simulink model "Model_6DOF_2021a"  (R2021b)
settings: Solver=FixedStepAuto  StartTime=0.0  StopTime=Tfin  FixedStep=0.05  RelTol=1e-3
values from neighbouring files (symbols this model uses):
  adap = 1    [ctrl_mode_param.m]
  Ba_0 = [0 0 0 0 0 0]    [ctrl_mode_param.m]
  Bv_0 = [tgt_speed 0 0 0 0 0]    [ctrl_mode_param.m]
  Bx_0 = [0 0 tgt_depth 0 0 0]    [ctrl_mode_param.m]
  check_angle = 10    [ctrl_mode_param.m]
  Cp = [Cpx' ; Cpy' ; Cpz']    [ctrl_mode_param.m]
  Cp_prime = Cp*Dm    [ctrl_mode_param.m]
  ctrl_mode = 5    [run.m]
  dX_imposed = 10    [ctrl_mode_param.m]
  Seastate = 5    [ctrl_mode_param.m]    (also in run.m = 0)
  tgt_depth = -50    [ctrl_mode_param.m]
  tgt_pitch = 0    [ctrl_mode_param.m]
  tgt_speed = -5    [ctrl_mode_param.m]
  tgt_sway = 0    [ctrl_mode_param.m]
  tgt_yaw = 0    [ctrl_mode_param.m]
undefined symbols (not defined in the file or in its folder): Bb, dA_BP1, dA_BP2, dA_Hull, dA_PH, dA_Sail, dA_SProot, dA_X1a, dA_X1b, dA_X2a, dA_X2b, dA_X3a, dA_X3b, dA_X4a, dA_X4b, Ixx, Ixy, Ixz, Iyy, Iyz, Izz, Mb, n_BP1, n_BP2, n_Hull, n_PH, n_Sail, n_SProot, n_X2a, n_X2b, n_X3a, n_X4a, n_X4b, nt_BP1, nt_BP2, nt_Hull, nt_PH, nt_Sail, nt_SProot, nt_X1a, nt_X1b, nt_X2a, nt_X2b, nt_X3a, nt_X3b, nt_X4a, nt_X4b, vt1_BP1, vt1_BP2, vt1_Hull, vt1_PH, vt1_Sail, vt1_SProot, vt1_X1a, vt1_X1b, vt1_X2a, vt1_X2b, vt1_X3a, vt1_X3b, vt1_X4a ... (+36)
libraries: simulink x19
(part 3 of 6)

== system Model_6DOF_2021a/HDM/HDM B3/M/Mdxi ==
  dX : Inport
  z : Inport  Port=2
  Demux6 : Demux  Outputs=5
  Gain{,1..4} (5 alike) : Gain
  Mux : Mux  Inputs=5
  ZudX1 q+1 : Lookup_n-D  BreakpointsForDimension1=[-30 -20 -10 0 10 20 30]  BreakpointsForDimension2=[-35.0624 -15.3724 -13.8724]  BreakpointsForDimension3=[-5.14444 -3.08666664 -1.54332]  Table=|  InternalRulePriority=Speed  RndMeth=Simplest  InputSameDT=on
      | reshape([0.000594819
      | 0.000394915
      | 0.000195011
      | -4.89222E-06
      | -0.000204796
      | -0.0004047
      | -0.000604603
      | 0.000596203
      | 0.000392018
      | 0.000187833
      | -1.6352E-05
      | -0.000220537
      | -0.000424722
      | -0.000628907
      | 0.000582351
      | 0.000381446
      | 0.000180542
      | -2.03625E-05
      | -0.000221267
      | -0.000422171
      | -0.000623076
      | ],[7,3])
      settings: InputPortMap=u0,u1
  ZudX1 q+2 : Lookup_n-D  BreakpointsForDimension1=[-30 -20 -10 0 10 20 30]  BreakpointsForDimension2=[-35.0624 -15.3724 -13.8724]  BreakpointsForDimension3=[-5.14444 -3.08666664 -1.54332]  Table=|  InternalRulePriority=Speed  RndMeth=Simplest  InputSameDT=on
      | reshape([0.000583784
      | 0.000394316
      | 0.000204847
      | 1.53782E-05
      | -0.000174091
      | -0.000363559
      | -0.000553028
      | 0.00056228
      | 0.000374724
      | 0.000187169
      | -3.86644E-07
      | -0.000187942
      | -0.000375498
      | -0.000563053
      | 0.000546298
      | 0.000362052
      | 0.000177806
      | -6.43933E-06
      | -0.000190685
      | -0.000374931
      | -0.000559176],[7,3])
      settings: InputPortMap=u0,u1
  ZudX1 q+3 : Lookup_n-D  BreakpointsForDimension1=[-30 -20 -10 0 10 20 30]  BreakpointsForDimension2=[-35.0624 -15.3724 -13.8724]  BreakpointsForDimension3=[-5.14444 -3.08666664 -1.54332]  Table=|  InternalRulePriority=Speed  RndMeth=Simplest  InputSameDT=on
      | reshape([-0.000586989
      | -0.000395541
      | -0.000204094
      | -1.26467E-05
      | 0.000178801
      | 0.000370248
      | 0.000561695
      | -0.000568868
      | -0.000379268
      | -0.000189669
      | -6.86388E-08
      | 0.000189531
      | 0.000379131
      | 0.000568731
      | -0.000565299
      | -0.000378949
      | -0.000192598
      | -6.24776E-06
      | 0.000180103
      | 0.000366453
      | 0.000552804],[7,3])
      settings: InputPortMap=u0,u1
  ZudX1 q+4 : Lookup_n-D  BreakpointsForDimension1=[-30 -20 -10 0 10 20 30]  BreakpointsForDimension2=[-35.0624 -15.3724 -13.8724]  BreakpointsForDimension3=[-5.14444 -3.08666664 -1.54332]  Table=|  InternalRulePriority=Speed  RndMeth=Simplest  InputSameDT=on
      | reshape([-0.000638396
      | -0.000426715
      | -0.000215035
      | -3.35454E-06
      | 0.000208326
      | 0.000420006
      | 0.000631687
      | -0.000598951
      | -0.000393944
      | -0.000188937
      | 1.60698E-05
      | 0.000221077
      | 0.000426084
      | 0.000631091
      | -0.000622514
      | -0.000421726
      | -0.000220939
      | -2.01522E-05
      | 0.000180635
      | 0.000381422
      | 0.000582209],[7,3])
      settings: InputPortMap=u0,u1
  ZudX1 q+5 : Lookup_n-D  BreakpointsForDimension1=[-30 -20 -10 0 10 20 30]  BreakpointsForDimension2=[-35.0624 -15.3724 -13.8724]  BreakpointsForDimension3=[-35.0624 -15.3724 -13.8724]  Table=|  InternalRulePriority=Speed  RndMeth=Simplest  InputSameDT=on
      | reshape([-0.000461714
      | -0.000296336
      | -0.000130959
      | 3.44194E-05
      | 0.000199797
      | 0.000365175
      | 0.000530553
      | -0.000503641
      | -0.000327652
      | -0.000151663
      | 2.43257E-05
      | 0.000200315
      | 0.000376303
      | 0.000552292
      | -0.000536558
      | -0.000356664
      | -0.00017677
      | 3.1235E-06
      | 0.000183017
      | 0.000362911
      | 0.000542805],[7,3])
      settings: InputPortMap=u0,u1
  MdX : Outport
  wires:
  Demux6/5 -> ZudX1 q+5/1
  Demux6/4 -> ZudX1 q+4/1
  Demux6/3 -> ZudX1 q+3/1
  Demux6/2 -> ZudX1 q+2/1
  ZudX1 q+4/1 -> Gain1/1
  ZudX1 q+3/1 -> Gain2/1
  ZudX1 q+2/1 -> Gain3/1
  ZudX1 q+1/1 -> Gain/1
  ZudX1 q+5/1 -> Gain4/1
  z/1 -> ZudX1 q+5/2, ZudX1 q+4/2, ZudX1 q+3/2, ZudX1 q+2/2, ZudX1 q+1/2
  Mux/1 -> MdX/1
  Demux6/1 -> ZudX1 q+1/1
  dX/1 -> Demux6/1
  Gain/1 -> Mux/1
  Gain3/1 -> Mux/2
  Gain2/1 -> Mux/3
  Gain1/1 -> Mux/4
  Gain4/1 -> Mux/5

== system Model_6DOF_2021a/HDM/HDM B3/N/NdXi ==
  dX : Inport
  z : Inport  Port=2
  Mux : Mux
  NdX1 : Lookup_n-D  BreakpointsForDimension1=[-10 0 10]  BreakpointsForDimension2=|  BreakpointsForDimension3=[-5.14444 -3.08666664 -1.54332]  Table=|  InternalRulePriority=Speed  RndMeth=Simplest  InputSameDT=on
      BreakpointsForDimension2=|
      | [-36.4062987
      | -18.4062987
      | -15.4062987
      | -13.9062987]
      Table=|
      | reshape([-8.13475E-05
      | -3.25752E-06
      | 6.9363E-05
      | -8.00129E-05
      | -1.7093E-06
      | 7.14001E-05
      | -6.46417E-05
      | -1.7093E-06
      | 8.57128E-05
      | -7.85432E-05
      | -1.19372E-08
      | 7.37459E-05],[3,4])
      settings: InputPortMap=u0,u1
  NdX2 : Lookup_n-D  BreakpointsForDimension1=[-10 0 10]  BreakpointsForDimension2=|  BreakpointsForDimension3=[-5.14444 -3.08666664 -1.54332]  Table=|  InternalRulePriority=Speed  RndMeth=Simplest  InputSameDT=on
      BreakpointsForDimension2=|
      | [-36.4062987
      | -18.4062987
      | -15.4062987
      | -13.9062987]
      Table=|
      | reshape([6.2278E-05
      | -3.5277E-06
      | -7.1028E-05
      | 5.9473E-05
      | -6.2352E-06
      | -7.5067E-05
      | 3.9525E-05
      | -6.2352E-06
      | -9.4282E-05
      | 5.5892E-05
      | -1.0640E-05
      | -8.2654E-05],[3,4])
      settings: InputPortMap=u0,u1
  NdX3 : Lookup_n-D  BreakpointsForDimension1=[-10 0 10]  BreakpointsForDimension2=|  BreakpointsForDimension3=[-5.14444 -3.08666664 -1.54332]  Table=|  InternalRulePriority=Speed  RndMeth=Simplest  InputSameDT=on
      BreakpointsForDimension2=|
      | [-36.4062987
      | -18.4062987
      | -15.4062987
      | -13.9062987]
      Table=|
      | reshape([8.96891E-05
      | 3.65995E-06
      | -8.07998E-05
      | 9.13096E-05
      | 6.34009E-06
      | -7.59117E-05
      | 0.000100356
      | 6.34009E-06
      | -4.56822E-05
      | 9.40576E-05
      | 1.06795E-05
      | -6.79415E-05],[3,4])
      settings: InputPortMap=u0,u1
  NdX4 : Lookup_n-D  BreakpointsForDimension1=[-10 0 10]  BreakpointsForDimension2=|  BreakpointsForDimension3=[-5.14444 -3.08666664 -1.54332]  Table=|  InternalRulePriority=Speed  RndMeth=Simplest  InputSameDT=on
      BreakpointsForDimension2=|
      | [-36.4062987
      | -18.4062987
      | -15.4062987
      | -13.9062987]
      Table=|
      | reshape([-7.16232E-05
      | 3.25314E-06
      | 8.32589E-05
      | -7.3213E-05
      | 1.68586E-06
      | 8.13825E-05
      | -8.66615E-05
      | 1.68586E-06
      | 6.54218E-05
      | -7.48528E-05
      | -6.7812E-08
      | 7.92559E-05],[3,4])
      settings: InputPortMap=u0,u1
  Selector1 : Selector  InputPortWidth=5  IndexOptions=Index vector (dialog)  Indices=2  OutputSizes=1
  Selector2 : Selector  InputPortWidth=5  IndexOptions=Index vector (dialog)  Indices=3  OutputSizes=1
  Selector3 : Selector  InputPortWidth=5  IndexOptions=Index vector (dialog)  Indices=4  OutputSizes=1
  Selector7 : Selector  InputPortWidth=5  IndexOptions=Index vector (dialog)  Indices=1  OutputSizes=1
  NdXi : Outport
  wires:
  dX/1 -> Selector3/1, Selector2/1, Selector1/1, Selector7/1
  Selector7/1 -> NdX1/1
  Mux/1 -> NdXi/1
  z/1 -> NdX4/2, NdX3/2, NdX2/2, NdX1/2
  NdX1/1 -> Mux/1
  NdX2/1 -> Mux/2
  NdX3/1 -> Mux/3
  NdX4/1 -> Mux/4
  Selector1/1 -> NdX2/1
  Selector2/1 -> NdX3/1
  Selector3/1 -> NdX4/1

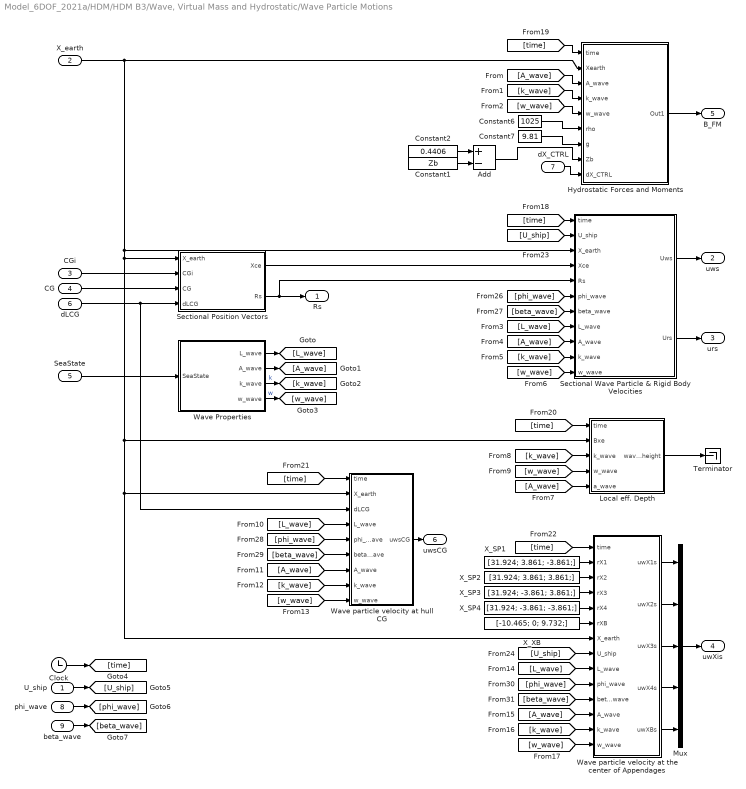
== system Model_6DOF_2021a/HDM/HDM B3/Wave, Virtual Mass and Hydrostatic/Wave Particle Motions ==
  U_ship : Inport
  X_earth : Inport  Port=2
  CGi : Inport  Port=3
  CG : Inport  Port=4
  SeaState : Inport  Port=5
  dLCG : Inport  Port=6
  dX_CTRL : Inport  Port=7
  phi_wave : Inport  Port=8
  beta_wave : Inport  Port=9
  Add : Sum  Inputs=+-
  Clock : Clock
  Constant1 : Constant  Value=Zb
  Constant2 : Constant  Value=0.4406
  Constant6 : Constant  Value=1025
  Constant7 : Constant  Value=9.81
  Hydrostatic Forces and Moments : Subsystem
  Local eff. Depth : MATLAB Function  TreatAsAtomicUnit=on
  Mux : Mux  Inputs=5
  Sectional Position Vectors : MATLAB Function  TreatAsAtomicUnit=on
  Sectional Wave Particle & Rigid Body Velocities : MATLAB Function  TreatAsAtomicUnit=on
  Terminator : Terminator
  Wave Properties : MATLAB Function  TreatAsAtomicUnit=on
  Wave particle velocity at hull CG : MATLAB Function  TreatAsAtomicUnit=on
  Wave particle velocity at the center of Appendages : MATLAB Function  TreatAsAtomicUnit=on
  X_SP1 : Constant  Value=[31.924; 3.861; -3.861;]
  X_SP2 : Constant  Value=[31.924; 3.861; 3.861;]
  X_SP3 : Constant  Value=[31.924; -3.861; 3.861;]
  X_SP4 : Constant  Value=[31.924; -3.861; -3.861;]
  X_XB : Constant  Value=[-10.465; 0; 9.732;]
  Rs : Outport
  uws : Outport  Port=2
  urs : Outport  Port=3
  uwXis : Outport  Port=4
  B_FM : Outport  Port=5
  uwsCG : Outport  Port=6
  wires:
  Sectional Position Vectors/2(Rs) -> Rs/1, Sectional Wave Particle & Rigid Body Velocities/5(Rs)
  SeaState/1 -> Wave Properties/1(SeaState)
  Sectional Position Vectors/1(Xce) -> Sectional Wave Particle & Rigid Body Velocities/4(Xce)
  X_earth/1 -> Wave particle velocity at hull CG/2(X_earth), Wave particle velocity at the center of Appendages/7(X_earth), Local eff. Depth/2(Bxe), Sectional Position Vectors/1(X_earth), Sectional Wave Particle & Rigid Body Velocities/3(X_earth), Hydrostatic Forces and Moments/2(Xearth)
  CGi/1 -> Sectional Position Vectors/2(CGi)
  CG/1 -> Sectional Position Vectors/3(CG)
  Sectional Wave Particle & Rigid Body Velocities/2(Urs) -> urs/1
  Sectional Wave Particle & Rigid Body Velocities/1(Uws) -> uws/1
  dLCG/1 -> Wave particle velocity at hull CG/3(dLCG), Sectional Position Vectors/4(dLCG)
  Local eff. Depth/1(wave_height) -> Terminator/1
  X_XB/1 -> Wave particle velocity at the center of Appendages/6(rXB)
  X_SP4/1 -> Wave particle velocity at the center of Appendages/5(rX4)
  X_SP3/1 -> Wave particle velocity at the center of Appendages/4(rX3)
  X_SP2/1 -> Wave particle velocity at the center of Appendages/3(rX2)
  X_SP1/1 -> Wave particle velocity at the center of Appendages/2(rX1)
  Wave particle velocity at the center of Appendages/1(uwX1s) -> Mux/1
  Wave particle velocity at the center of Appendages/2(uwX2s) -> Mux/2
  Wave particle velocity at the center of Appendages/3(uwX3s) -> Mux/3
  Wave particle velocity at the center of Appendages/4(uwX4s) -> Mux/4
  Wave particle velocity at the center of Appendages/5(uwXBs) -> Mux/5
  Mux/1 -> uwXis/1
  Wave particle velocity at hull CG/1(uwsCG) -> uwsCG/1
  Hydrostatic Forces and Moments/1(Out1) -> B_FM/1
  Constant6/1 -> Hydrostatic Forces and Moments/6(rho)
  Constant7/1 -> Hydrostatic Forces and Moments/7(g)
  Add/1 -> Hydrostatic Forces and Moments/8(Zb)
  Constant2/1 -> Add/1
  Constant1/1 -> Add/2
  dX_CTRL/1 -> Hydrostatic Forces and Moments/9(dX_CTRL)
  Wave Properties/1(L_wave) -> [L_wave]
  Wave Properties/2(A_wave) -> [A_wave]
  Wave Properties/3(k_wave) -> [k_wave]  "k"
  Wave Properties/4(w_wave) -> [w_wave]  "w"
  [A_wave] -> Hydrostatic Forces and Moments/3(A_wave)
  [k_wave] -> Hydrostatic Forces and Moments/4(k_wave)
  [w_wave] -> Hydrostatic Forces and Moments/5(w_wave)
  [L_wave] -> Sectional Wave Particle & Rigid Body Velocities/8(L_wave)
  [A_wave] -> Sectional Wave Particle & Rigid Body Velocities/9(A_wave)
  [k_wave] -> Sectional Wave Particle & Rigid Body Velocities/10(k_wave)
  [w_wave] -> Sectional Wave Particle & Rigid Body Velocities/11(w_wave)
  [k_wave] -> Local eff. Depth/3(k_wave)
  [A_wave] -> Local eff. Depth/5(a_wave)
  [w_wave] -> Local eff. Depth/4(w_wave)
  [L_wave] -> Wave particle velocity at hull CG/4(L_wave)
  [A_wave] -> Wave particle velocity at hull CG/7(A_wave)
  [k_wave] -> Wave particle velocity at hull CG/8(k_wave)
  [w_wave] -> Wave particle velocity at hull CG/9(w_wave)
  [L_wave] -> Wave particle velocity at the center of Appendages/9(L_wave)
  [A_wave] -> Wave particle velocity at the center of Appendages/12(A_wave)
  [k_wave] -> Wave particle velocity at the center of Appendages/13(k_wave)
  [w_wave] -> Wave particle velocity at the center of Appendages/14(w_wave)
  Clock/1 -> [time]
  [time] -> Sectional Wave Particle & Rigid Body Velocities/1(time)
  [time] -> Hydrostatic Forces and Moments/1(time)
  [time] -> Local eff. Depth/1(time)
  [time] -> Wave particle velocity at hull CG/1(time)
  [time] -> Wave particle velocity at the center of Appendages/1(time)
  U_ship/1 -> [U_ship]
  [U_ship] -> Sectional Wave Particle & Rigid Body Velocities/2(U_ship)
  [U_ship] -> Wave particle velocity at the center of Appendages/8(U_ship)
  phi_wave/1 -> [phi_wave]
  beta_wave/1 -> [beta_wave]
  [phi_wave] -> Sectional Wave Particle & Rigid Body Velocities/6(phi_wave)
  [beta_wave] -> Sectional Wave Particle & Rigid Body Velocities/7(beta_wave)
  [phi_wave] -> Wave particle velocity at hull CG/5(phi_wave)
  [beta_wave] -> Wave particle velocity at hull CG/6(beta_wave)
  [phi_wave] -> Wave particle velocity at the center of Appendages/10(phi_wave)
  [beta_wave] -> Wave particle velocity at the center of Appendages/11(beta_wave)

== system Model_6DOF_2021a/HDM/HDM B3/X/X'dXi ==
  UeX : Inport
  dXeff : Inport  Port=2
  Gain : Gain  Gain=-1
  Gain{4..7} (4 alike) : Gain
  Mux : Mux  Inputs=5
  Saturation6 : Saturate  UpperLimit=-1.543332  LowerLimit=-5.14444
  Selector10 : Selector  InputPortWidth=5  IndexOptions=Index vector (dialog)  Indices=4  OutputSizes=1
  Selector11 : Selector  InputPortWidth=5  IndexOptions=Index vector (dialog)  Indices=4  OutputSizes=1
  Selector12 : Selector  InputPortWidth=5  IndexOptions=Index vector (dialog)  Indices=5  OutputSizes=1
  Selector2 : Selector  InputPortWidth=5  IndexOptions=Index vector (dialog)  Indices=5  OutputSizes=1
  Selector4 : Selector  InputPortWidth=5  IndexOptions=Index vector (dialog)  Indices=1  OutputSizes=1
  Selector5 : Selector  InputPortWidth=5  IndexOptions=Index vector (dialog)  Indices=1  OutputSizes=1
  Selector6 : Selector  InputPortWidth=5  IndexOptions=Index vector (dialog)  Indices=2  OutputSizes=1
  Selector7 : Selector  InputPortWidth=5  IndexOptions=Index vector (dialog)  Indices=2  OutputSizes=1
  Selector8 : Selector  InputPortWidth=5  IndexOptions=Index vector (dialog)  Indices=3  OutputSizes=1
  Selector9 : Selector  InputPortWidth=5  IndexOptions=Index vector (dialog)  Indices=3  OutputSizes=1
  To Workspace : ToWorkspace  VariableName=UeX  SaveFormat=Timeseries  SampleTime=-1
  XudX1 : Lookup_n-D  BreakpointsForDimension1=[-30 -20 -10 0 10 20 30]  BreakpointsForDimension2=|  Table=|  InternalRulePriority=Speed  RndMeth=Simplest  InputSameDT=on
      BreakpointsForDimension2=|
      | [-7.716666
      | -5.144444
      | -3.0866664
      | -1.5433332
      | ]
      Table=|
      | reshape([3.2151E-04
      | 1.4055E-04
      | 2.3723E-05
      | -2.9685E-05
      | 2.3777E-05
      | 1.3375E-04
      | 3.3722E-04
      | 1.6076E-04
      | 7.0275E-05
      | 1.1862E-05
      | -1.4843E-05
      | 1.1889E-05
      | 6.6875E-05
      | 1.6861E-04
      | 1.6698E-04
      | 6.8790E-05
      | 1.2322E-05
      | -1.4312E-05
      | 1.2274E-05
      | 6.7265E-05
      | 1.7083E-04
      | 3.4224E-04
      | 1.3333E-04
      | 2.5937E-05
      | -6.5668E-05
      | 2.5937E-05
      | 1.3102E-04
      | 3.4214E-04
      | ],[7,4])
      settings: InputPortMap=u0,u1
  XudX2 : Lookup_n-D  BreakpointsForDimension1=[-30 -20 -10 0 10 20 30]  BreakpointsForDimension2=|  Table=|  InternalRulePriority=Speed  RndMeth=Simplest  InputSameDT=on
      BreakpointsForDimension2=|
      | [-7.716666
      | -5.144444
      | -3.0866664
      | -1.5433332
      | ]
      Table=|
      | reshape([2.9233E-04
      | 1.3189E-04
      | 2.3224E-05
      | -2.9022E-05
      | 1.9675E-05
      | 1.4726E-04
      | 3.7676E-04
      | 1.4617E-04
      | 6.5945E-05
      | 1.1612E-05
      | -1.4511E-05
      | 9.8375E-06
      | 7.3630E-05
      | 1.8838E-04
      | 1.7319E-04
      | 6.7285E-05
      | 1.2060E-05
      | -2.5958E-05
      | 1.0337E-05
      | 7.6660E-05
      | 1.8963E-04
      | 3.4748E-04
      | 1.3335E-04
      | 2.2395E-05
      | -2.6403E-05
      | 2.2395E-05
      | 1.5181E-04
      | 3.8598E-04
      | ],[7,4])
      settings: InputPortMap=u0,u1
  XudX3 : Lookup_n-D  BreakpointsForDimension1=[-30 -20 -10 0 10 20 30]  BreakpointsForDimension2=|  Table=|  InternalRulePriority=Speed  RndMeth=Simplest  InputSameDT=on
      BreakpointsForDimension2=|
      | [-7.716666
      | -5.144444
      | -3.0866664
      | -1.5433332
      | ]
      Table=|
      | reshape([3.5642E-04
      | 1.5674E-04
      | 2.5449E-05
      | -2.9060E-05
      | 2.6726E-05
      | 1.6225E-04
      | 3.1115E-04
      | 1.7821E-04
      | 7.8370E-05
      | 1.2725E-05
      | -1.4530E-05
      | 1.3363E-05
      | 8.1125E-05
      | 1.5558E-04
      | 1.9053E-04
      | 8.0600E-05
      | 1.2911E-05
      | -1.3998E-05
      | 1.3672E-05
      | 7.4645E-05
      | 1.6290E-04
      | 3.8447E-04
      | 1.4526E-04
      | 2.7824E-05
      | -2.6434E-05
      | 2.7824E-05
      | 1.5039E-04
      | 3.2499E-04
      | ],[7,4])
      settings: InputPortMap=u0,u1
  XudX4 : Lookup_n-D  BreakpointsForDimension1=[-30 -20 -10 0 10 20 30]  BreakpointsForDimension2=|  Table=|  InternalRulePriority=Speed  RndMeth=Simplest  InputSameDT=on
      BreakpointsForDimension2=|
      | [-7.716666
      | -5.144444
      | -3.0866664
      | -1.5433332
      | ]
      Table=|
      | reshape([3.4525E-04
      | 1.3840E-04
      | 2.4668E-05
      | -2.9702E-05
      | 2.4205E-05
      | 1.2737E-04
      | 3.2790E-04
      | 1.7263E-04
      | 6.9200E-05
      | 1.2334E-05
      | -1.4851E-05
      | 1.2103E-05
      | 6.3685E-05
      | 1.6395E-04
      | 1.7298E-04
      | 6.9435E-05
      | 1.2696E-05
      | -1.4315E-05
      | 1.2608E-05
      | 6.9175E-05
      | 1.6779E-04
      | 3.3803E-04
      | 1.5513E-04
      | 2.6677E-05
      | -2.7052E-05
      | 2.6677E-05
      | 1.3644E-04
      | 3.3780E-04
      | ],[7,4])
      settings: InputPortMap=u0,u1
  XudXB : Lookup_n-D  BreakpointsForDimension1=[-30 -20 -10 0 10 20 30]  BreakpointsForDimension2=[-5.14444 -3.08666664 -1.54332]  Table=|  InternalRulePriority=Speed  RndMeth=Simplest  InputSameDT=on
      | reshape([6.9060E-04
      | 3.9256E-04
      | 1.5651E-04
      | 0.0000E+00
      | 1.1449E-04
      | 4.2412E-04
      | 5.7370E-04
      | 6.4542E-04
      | 3.9138E-04
      | 1.5593E-04
      | 0.0000E+00
      | 1.1381E-04
      | 4.1205E-04
      | 5.6813E-04
      | 6.5675E-04
      | 3.9410E-04
      | 1.1271E-04
      | 0.0000E+00
      | 1.1271E-04
      | 4.2649E-04
      | 5.7604E-04
      | ],[7,3])
      settings: InputPortMap=u0,u1
  Out1 : Outport
  wires:
  Selector2/1 -> XudXB/1
  XudX4/1 -> Gain7/1
  XudX3/1 -> Gain5/1
  XudX2/1 -> Gain6/1
  XudX1/1 -> Gain4/1
  Mux/1 -> Out1/1
  dXeff/1 -> Selector2/1, Selector10/1, Selector8/1, Selector6/1, Selector4/1
  Selector4/1 -> XudX1/1
  Selector5/1 -> XudX1/2
  Selector6/1 -> XudX2/1
  Selector7/1 -> XudX2/2
  Selector8/1 -> XudX3/1
  Selector9/1 -> XudX3/2
  UeX/1 -> Gain/1
  Selector11/1 -> XudX4/2
  Selector10/1 -> XudX4/1
  Selector12/1 -> XudXB/2
  Gain4/1 -> Mux/1
  Gain6/1 -> Mux/2
  Gain5/1 -> Mux/3
  Gain7/1 -> Mux/4
  XudXB/1 -> Mux/5
  Gain/1 -> To Workspace/1, Saturation6/1
  Saturation6/1 -> Selector11/1, Selector12/1, Selector9/1, Selector7/1, Selector5/1

== system Model_6DOF_2021a/HDM/HDM B3/Y/YdXi ==
  dX : Inport
  z : Inport  Port=2
  Mux : Mux
  Selector1 : Selector  InputPortWidth=5  IndexOptions=Index vector (dialog)  Indices=2  OutputSizes=1
  Selector2 : Selector  InputPortWidth=5  IndexOptions=Index vector (dialog)  Indices=3  OutputSizes=1
  Selector3 : Selector  InputPortWidth=5  IndexOptions=Index vector (dialog)  Indices=4  OutputSizes=1
  Selector7 : Selector  InputPortWidth=5  IndexOptions=Index vector (dialog)  Indices=1  OutputSizes=1
  YdX1 : Lookup_n-D  BreakpointsForDimension1=[-10 0 10]  BreakpointsForDimension2=|  BreakpointsForDimension3=[-5.14444 -3.08666664 -1.54332]  Table=|  InternalRulePriority=Speed  RndMeth=Simplest  InputSameDT=on
      BreakpointsForDimension2=|
      | [-36.4062987
      | -18.4062987
      | -15.4062987
      | -13.9062987]
      Table=|
      | reshape([-1.8282E-04
      | -6.0037E-06
      | 1.6496E-04
      | -1.7978E-04
      | -2.4314E-06
      | 1.6969E-04
      | -1.4480E-04
      | -2.4314E-06
      | 2.0267E-04
      | -1.7641E-04
      | 1.4850E-06
      | 1.7514E-04],[3,4])
      settings: InputPortMap=u0,u1
  YdX2 : Lookup_n-D  BreakpointsForDimension1=[-10 0 10]  BreakpointsForDimension2=|  BreakpointsForDimension3=[-5.14444 -3.08666664 -1.54332]  Table=|  InternalRulePriority=Speed  RndMeth=Simplest  InputSameDT=on
      BreakpointsForDimension2=|
      | [-36.4062987
      | -18.4062987
      | -15.4062987
      | -13.9062987]
      Table=|
      | reshape([1.4857E-04
      | -6.6611E-06
      | -1.5932E-04
      | 1.4200E-04
      | -1.2968E-05
      | -1.6860E-04
      | 9.4982E-05
      | -1.2968E-05
      | -2.1344E-04
      | 1.3366E-04
      | -2.3176E-05
      | -1.8599E-04],[3,4])
      settings: InputPortMap=u0,u1
  YdX3 : Lookup_n-D  BreakpointsForDimension1=[-10 0 10]  BreakpointsForDimension2=|  BreakpointsForDimension3=[-5.14444 -3.08666664 -1.54332]  Table=|  InternalRulePriority=Speed  RndMeth=Simplest  InputSameDT=on
      BreakpointsForDimension2=|
      | [-36.4062987
      | -18.4062987
      | -15.4062987
      | -13.9062987]
      Table=|
      | reshape([2.0207E-04
      | 6.9701E-06
      | -1.9141E-04
      | 2.0588E-04
      | 1.3213E-05
      | -1.8007E-04
      | 2.2753E-04
      | 1.3213E-05
      | -1.0937E-04
      | 2.1222E-04
      | 2.3270E-05
      | -1.6161E-04],[3,4])
      settings: InputPortMap=u0,u1
  YdX4 : Lookup_n-D  BreakpointsForDimension1=[-10 0 10]  BreakpointsForDimension2=|  BreakpointsForDimension3=[-5.14444 -3.08666664 -1.54332]  Table=|  InternalRulePriority=Speed  RndMeth=Simplest  InputSameDT=on
      BreakpointsForDimension2=|
      | [-36.4062987
      | -18.4062987
      | -15.4062987
      | -13.9062987]
      Table=|
      | reshape([-1.7022E-04
      | 5.9932E-06
      | 1.8722E-04
      | -1.7390E-04
      | 2.3770E-06
      | 1.8293E-04
      | -2.0489E-04
      | 2.3770E-06
      | 1.4658E-04
      | -1.7771E-04
      | -1.6689E-06
      | 1.7805E-04],[3,4])
      settings: InputPortMap=u0,u1
  YdX : Outport
  wires:
  Mux/1 -> YdX/1
  z/1 -> YdX4/2, YdX3/2, YdX2/2, YdX1/2
  YdX1/1 -> Mux/1
  YdX2/1 -> Mux/2
  YdX3/1 -> Mux/3
  YdX4/1 -> Mux/4
  Selector7/1 -> YdX1/1
  dX/1 -> Selector2/1, Selector3/1, Selector1/1, Selector7/1
  Selector3/1 -> YdX4/1
  Selector2/1 -> YdX3/1
  Selector1/1 -> YdX2/1

== system Model_6DOF_2021a/HDM/HDM B3/Z/ZdXi ==
  dX : Inport
  z : Inport  Port=2
  Demux6 : Demux  Outputs=5
  Mux : Mux  Inputs=5
  ZudX1 q+10 : Lookup_n-D  BreakpointsForDimension1=[-30 -20 -10 0 10 20 30]  BreakpointsForDimension2=[-35.0624 -15.3724 -13.8724]  BreakpointsForDimension3=[-35.0624 -15.3724 -13.8724]  Table=|  InternalRulePriority=Speed  RndMeth=Simplest  InputSameDT=on
      | reshape([-0.003226964
      | -0.002116041
      | -0.001005119
      | 0.000105803
      | 0.001216725
      | 0.002327647
      | 0.003438569
      | -0.003036597
      | -0.001876165
      | -0.000715732
      | 0.0004447
      | 0.001605132
      | 0.002765565
      | 0.003925997
      | -0.003676642
      | -0.002490275
      | -0.001303908
      | -0.000117541
      | 0.001068826
      | 0.002255193
      | 0.00344156],[7,3])
      settings: InputPortMap=u0,u1
  ZudX1 q+6 : Lookup_n-D  BreakpointsForDimension1=[-30 -20 -10 0 10 20 30]  BreakpointsForDimension2=[-35.0624 -15.3724 -13.8724]  BreakpointsForDimension3=[-5.14444 -3.08666664 -1.54332]  Table=|  InternalRulePriority=Speed  RndMeth=Simplest  InputSameDT=on
      | reshape([-0.001383757
      | -0.000911
      | -0.000438243
      | 3.45135E-05
      | 0.00050727
      | 0.000980027
      | 0.001452784
      | -0.001383757
      | -0.000911
      | -0.000438243
      | 3.45135E-05
      | 0.00050727
      | 0.000980027
      | 0.001452784
      | -0.001353354
      | -0.000887631
      | -0.000421908
      | 4.38143E-05
      | 0.000509537
      | 0.00097526
      | 0.001440982],[7,3])
      settings: InputPortMap=u0,u1
  ZudX1 q+7 : Lookup_n-D  BreakpointsForDimension1=[-30 -20 -10 0 10 20 30]  BreakpointsForDimension2=[-35.0624 -15.3724 -13.8724]  BreakpointsForDimension3=[-5.14444 -3.08666664 -1.54332]  Table=|  InternalRulePriority=Speed  RndMeth=Simplest  InputSameDT=on
      | reshape([-0.001358511
      | -0.00091651
      | -0.000474508
      | -3.25062E-05
      | 0.000409495
      | 0.000851497
      | 0.001293499
      | -0.001303275
      | -0.00086798
      | -0.000432686
      | 2.60877E-06
      | 0.000437903
      | 0.000873198
      | 0.001308493
      | -0.001263287
      | -0.000836064
      | -0.00040884
      | 1.83841E-05
      | 0.000445608
      | 0.000872832
      | 0.001300056],[7,3])
      settings: InputPortMap=u0,u1
  ZudX1 q+8 : Lookup_n-D  BreakpointsForDimension1=[-30 -20 -10 0 10 20 30]  BreakpointsForDimension2=[-35.0624 -15.3724 -13.8724]  BreakpointsForDimension3=[-5.14444 -3.08666664 -1.54332]  Table=|  InternalRulePriority=Speed  RndMeth=Simplest  InputSameDT=on
      | reshape([0.001309084
      | 0.000864124
      | 0.000419163
      | -2.5798E-05
      | -0.000470759
      | -0.000915719
      | -0.00136068
      | 0.001321953
      | 0.000882434
      | 0.000442915
      | 3.39516E-06
      | -0.000436124
      | -0.000875644
      | -0.001315163
      | 0.001313186
      | 0.000881448
      | 0.000449709
      | 1.79712E-05
      | -0.000413767
      | -0.000845505
      | -0.001277243],[7,3])
      settings: InputPortMap=u0,u1
  ZudX1 q+9 : Lookup_n-D  BreakpointsForDimension1=[-30 -20 -10 0 10 20 30]  BreakpointsForDimension2=[-35.0624 -15.3724 -13.8724]  BreakpointsForDimension3=[-5.14444 -3.08666664 -1.54332]  Table=|  InternalRulePriority=Speed  RndMeth=Simplest  InputSameDT=on
      | reshape([0.001464336
      | 0.000977857
      | 0.000491377
      | 4.89775E-06
      | -0.000481582
      | -0.000968061
      | -0.00145454
      | 0.001455937
      | 0.00098192
      | 0.000507903
      | 3.38863E-05
      | -0.00044013
      | -0.000914147
      | -0.001388164
      | 0.001460604
      | 0.00098818
      | 0.000515756
      | 4.33325E-05
      | -0.000429091
      | -0.000901515
      | -0.001373939],[7,3])
      settings: InputPortMap=u0,u1
  ZdX : Outport
  wires:
  ZudX1 q+9/1 -> Mux/4
  ZudX1 q+8/1 -> Mux/3
  ZudX1 q+7/1 -> Mux/2
  ZudX1 q+6/1 -> Mux/1
  ZudX1 q+10/1 -> Mux/5
  z/1 -> ZudX1 q+9/2, ZudX1 q+10/2, ZudX1 q+8/2, ZudX1 q+7/2, ZudX1 q+6/2
  Demux6/5 -> ZudX1 q+10/1
  Mux/1 -> ZdX/1
  Demux6/1 -> ZudX1 q+6/1
  Demux6/2 -> ZudX1 q+7/1
  Demux6/4 -> ZudX1 q+9/1
  dX/1 -> Demux6/1
  Demux6/3 -> ZudX1 q+8/1

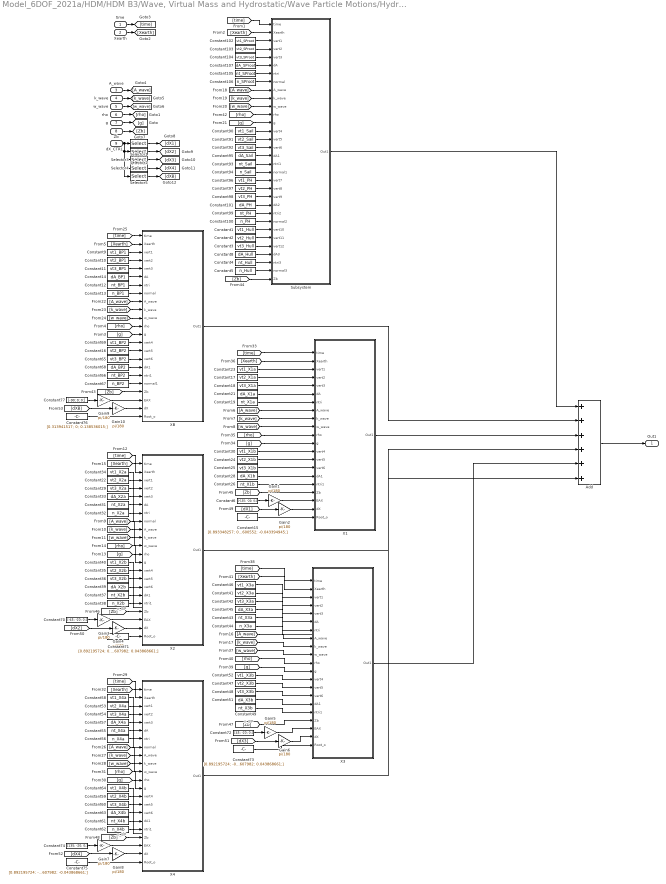
== system Model_6DOF_2021a/HDM/HDM B3/Wave, Virtual Mass and Hydrostatic/Wave Particle Motions/Hydrostatic Forces and Moments ==
  note: n_BP
  note: n_BP
  note: n_BP
  time : Inport
  Xearth : Inport  Port=2
  A_wave : Inport  Port=3
  k_wave : Inport  Port=4
  w_wave : Inport  Port=5
  rho : Inport  Port=6
  g : Inport  Port=7
  Zb : Inport  Port=8
  dX_CTRL : Inport  Port=9
  Add : Sum  Inputs=6
  Constant1 : Constant  Value=vt1_Hull
  Constant10 : Constant  Value=vt2_BP1
  Constant100 : Constant  Value=n_PH
  Constant101 : Constant  Value=dA_PH
  Constant102 : Constant  Value=vt1_SProot
  Constant103 : Constant  Value=vt2_SProot
  Constant104 : Constant  Value=vt3_SProot
  Constant105 : Constant  Value=nt_SProot
  Constant106 : Constant  Value=n_SProot
  Constant107 : Constant  Value=dA_SProot
  Constant11 : Constant  Value=vt3_BP1
  Constant12 : Constant  Value=nt_BP1
  Constant13 : Constant  Value=n_BP1
  Constant14 : Constant  Value=dA_BP1
  Constant15 : Constant  Value=|
      | [0.893348257;
      | 0.043600552;
      | -0.043394945;]
  Constant16 : Constant  Value=vt2_BP2
  Constant17 : Constant  Value=vt2_X1a
  Constant18 : Constant  Value=vt3_X1a
  Constant19 : Constant  Value=nt_X1a
  Constant2 : Constant  Value=vt2_Hull
  Constant21 : Constant  Value=dA_X1a
  Constant22 : Constant  Value=vt2_X2a
  Constant23 : Constant  Value=vt1_X1a
  Constant24 : Constant  Value=vt2_X1b
  Constant25 : Constant  Value=vt3_X1b
  Constant26 : Constant  Value=nt_X1b
  Constant28 : Constant  Value=dA_X1b
  Constant29 : Constant  Value=vt3_X2a
  Constant3 : Constant  Value=vt3_Hull
  Constant30 : Constant  Value=vt1_X1b
  Constant31 : Constant  Value=nt_X2a
  Constant32 : Constant  Value=n_X2a
  Constant33 : Constant  Value=dA_X2a
  Constant34 : Constant  Value=vt1_X2a
  Constant35 : Constant  Value=vt2_X2b
  Constant36 : Constant  Value=vt3_X2b
  Constant37 : Constant  Value=nt_X2b
  Constant38 : Constant  Value=n_X2b
  Constant39 : Constant  Value=dA_X2b
  Constant4 : Constant  Value=nt_Hull
  Constant40 : Constant  Value=vt1_X2b
  Constant41 : Constant  Value=vt2_X3a
  Constant42 : Constant  Value=vt3_X3a
  Constant43 : Constant  Value=nt_X3a
  Constant44 : Constant  Value=n_X3a
  Constant45 : Constant  Value=dA_X3a
  Constant46 : Constant  Value=vt1_X3a
  Constant47 : Constant  Value=vt2_X3b
  Constant48 : Constant  Value=vt3_X3b
  Constant49 : Constant  Value=nt_X3b
  Constant5 : Constant  Value=n_Hull
  Constant51 : Constant  Value=dA_X3b
  Constant52 : Constant  Value=vt1_X3b
  Constant53 : Constant  Value=vt2_X4a
  Constant54 : Constant  Value=vt3_X4a
  Constant55 : Constant  Value=nt_X4a
  Constant56 : Constant  Value=n_X4a
  Constant57 : Constant  Value=dA_X4a
  Constant58 : Constant  Value=vt1_X4a
  Constant59 : Constant  Value=vt2_X4b
  Constant6 : Constant  Value=[-135; -20; 0;]
  Constant60 : Constant  Value=vt3_X4b
  Constant61 : Constant  Value=nt_X4b
  Constant62 : Constant  Value=n_X4b
  Constant63 : Constant  Value=dA_X4b
  Constant64 : Constant  Value=vt1_X4b
  Constant65 : Constant  Value=vt3_BP2
  Constant66 : Constant  Value=nt_BP2
  Constant67 : Constant  Value=n_BP2
  Constant68 : Constant  Value=dA_BP2
  Constant69 : Constant  Value=vt1_BP2
  Constant70 : Constant  Value=[-45; -20; 0;]
  Constant71 : Constant  Value=|
      | [0.892195724;
      | 0.043607982;
      | 0.043868661;]
  Constant72 : Constant  Value=[45; -20; 0;]
  Constant73 : Constant  Value=|
      | [0.892195724;
      | -0.043607982;
      | 0.043868661;]
  Constant74 : Constant  Value=[135; -20; 0;]
  Constant75 : Constant  Value=|
      | [0.892195724;
      | -0.043607982;
      | -0.043868661;]
  Constant76 : Constant  Value=|
      | [0.313941517;
      | 0;
      | 0.138536015;]
  Constant77 : Constant  Value=[-90; 0; 0;]
  Constant8 : Constant  Value=dA_Hull
  Constant9 : Constant  Value=vt1_BP1
  Constant90 : Constant  Value=vt1_Sail
  Constant91 : Constant  Value=vt2_Sail
  Constant92 : Constant  Value=vt3_Sail
  Constant93 : Constant  Value=nt_Sail
  Constant94 : Constant  Value=n_Sail
  Constant95 : Constant  Value=dA_Sail
  Constant96 : Constant  Value=vt1_PH
  Constant97 : Constant  Value=vt2_PH
  Constant98 : Constant  Value=vt3_PH
  Constant99 : Constant  Value=nt_PH
  Gain{1..10} (10 alike) : Gain  Gain=pi/180
  Selector1 : Selector  InputPortWidth=5  IndexOptions=Index vector (dialog)  Indices=1  OutputSizes=1
  Selector2 : Selector  InputPortWidth=5  IndexOptions=Index vector (dialog)  Indices=2  OutputSizes=1
  Selector3 : Selector  InputPortWidth=5  IndexOptions=Index vector (dialog)  Indices=3  OutputSizes=1
  Selector4 : Selector  InputPortWidth=5  IndexOptions=Index vector (dialog)  Indices=4  OutputSizes=1
  Selector5 : Selector  InputPortWidth=5  IndexOptions=Index vector (dialog)  Indices=5  OutputSizes=1
  Subsystem : Subsystem
  X1 : Subsystem
  X2 : Subsystem
  X3 : Subsystem
  X4 : Subsystem
  XB : Subsystem
  Out1 : Outport
  wires:
  time/1 -> [time]
  Xearth/1 -> [Xearth]
  A_wave/1 -> [A_wave]
  k_wave/1 -> [k_wave]
  w_wave/1 -> [w_wave]
  rho/1 -> [rho]
  g/1 -> [g]
  Constant94/1 -> Subsystem/19(normal1)
  Constant61/1 -> X4/18(ntri1)
  Constant57/1 -> X4/6(dA)
  [Zb] -> X4/19(Zb)
  [Zb] -> X3/18(Zb)
  Constant101/1 -> Subsystem/23(dA2)
  Constant16/1 -> XB/15(vert5)
  [Zb] -> X1/18(Zb)
  [Zb] -> X2/19(Zb)
  Constant98/1 -> Subsystem/22(vert9)
  Constant99/1 -> Subsystem/24(ntri2)
  Constant37/1 -> X2/18(ntri1)
  [Zb] -> XB/20(Zb)
  [time] -> X3/1(time)
  [Xearth] -> X1/2(Xearth)
  [w_wave] -> Subsystem/11(w_wave)
  Constant93/1 -> Subsystem/18(ntri1)
  [g] -> X2/13(g)
  Constant28/1 -> X1/16(dA1)
  [w_wave] -> X3/10(w_wave)
  Constant8/1 -> Subsystem/29(dA3)
  Constant95/1 -> Subsystem/17(dA1)
  [A_wave] -> X4/9(A_wave)
  Constant33/1 -> X2/6(dA)
  [rho] -> X4/12(rho)
  [time] -> Subsystem/1(time)
  Constant48/1 -> X3/15(vert6)
  [rho] -> Subsystem/12(rho)
  Constant60/1 -> X4/16(vert6)
  [k_wave] -> Subsystem/10(k_wave)
  Constant19/1 -> X1/7(ntri)
  [g] -> Subsystem/13(g)
  Constant102/1 -> Subsystem/3(vert1)
  Constant106/1 -> Subsystem/8(normal)
  [Xearth] -> Subsystem/2(Xearth)
  Constant107/1 -> Subsystem/6(dA)
  Constant105/1 -> Subsystem/7(ntri)
  [g] -> X4/13(g)
  Constant11/1 -> XB/5(vert3)
  Constant34/1 -> X2/3(vert1)
  Constant63/1 -> X4/17(dA1)
  [A_wave] -> X1/8(A_wave)
  Constant41/1 -> X3/4(vert2)
  [k_wave] -> X2/10(k_wave)
  Constant22/1 -> X2/4(vert2)
  Constant49/1 -> X3/17(ntri1)
  [Xearth] -> XB/2(Xearth)
  [rho] -> X2/12(rho)
  [rho] -> X3/11(rho)
  Constant55/1 -> X4/7(ntri)
  Constant45/1 -> X3/6(dA)
  Constant40/1 -> X2/14(vert4)
  Constant18/1 -> X1/5(vert3)
  [g] -> X1/12(g)
  Constant35/1 -> X2/15(vert5)
  Constant39/1 -> X2/17(dA1)
  Constant32/1 -> X2/8(normal)
  Constant47/1 -> X3/14(vert5)
  [w_wave] -> X4/11(w_wave)
  Constant44/1 -> ?
  [k_wave] -> X1/9(k_wave)
  Constant53/1 -> X4/4(vert2)
  [w_wave] -> XB/11(w_wave)
  [Xearth] -> X2/2(Xearth)
  [time] -> XB/1(time)
  [rho] -> XB/12(rho)
  Constant4/1 -> Subsystem/30(ntri3)
  Constant59/1 -> X4/15(vert5)
  Constant51/1 -> X3/16(dA1)
  Constant52/1 -> X3/13(vert4)
  Constant14/1 -> XB/6(dA)
  [Xearth] -> X3/2(Xearth)
  Constant25/1 -> X1/15(vert6)
  Constant67/1 -> XB/19(normal1)
  [Zb] -> Subsystem/32(Zb)
  Constant65/1 -> XB/16(vert6)
  Constant104/1 -> Subsystem/5(vert3)
  Constant13/1 -> XB/8(normal)
  Constant69/1 -> XB/14(vert4)
  Constant43/1 -> X3/7(ntri)
  [k_wave] -> X3/9(k_wave)
  [A_wave] -> X2/9(A_wave)
  Constant17/1 -> X1/4(vert2)
  [k_wave] -> XB/10(k_wave)
  Constant68/1 -> XB/17(dA1)
  Constant46/1 -> X3/3(vert1)
  Constant23/1 -> X1/3(vert1)
  Constant9/1 -> XB/3(vert1)
  Constant62/1 -> ?
  [A_wave] -> XB/9(A_wave)
  Constant26/1 -> X1/17(ntri1)
  Constant56/1 -> X4/8(normal)
  Constant24/1 -> X1/14(vert5)
  Constant12/1 -> XB/7(ntri)
  [g] -> X3/12(g)
  [w_wave] -> X1/10(w_wave)
  Constant100/1 -> Subsystem/25(normal2)
  Constant92/1 -> Subsystem/16(vert6)
  Constant30/1 -> X1/13(vert4)
  [time] -> X2/1(time)
  [rho] -> X1/11(rho)
  Constant91/1 -> Subsystem/15(vert5)
  [time] -> X1/1(time)
  Constant1/1 -> Subsystem/26(vert10)
  Constant31/1 -> X2/7(ntri)
  [w_wave] -> X2/11(w_wave)
  Constant21/1 -> X1/6(dA)
  Constant90/1 -> Subsystem/14(vert4)
  Constant96/1 -> Subsystem/20(vert7)
  Constant36/1 -> X2/16(vert6)
  Constant29/1 -> X2/5(vert3)
  [Xearth] -> X4/2(Xearth)
  Constant64/1 -> X4/14(vert4)
  Constant97/1 -> Subsystem/21(vert8)
  Constant2/1 -> Subsystem/27(vert11)
  Constant66/1 -> XB/18(ntri1)
  Constant54/1 -> X4/5(vert3)
  Constant38/1 -> ?
  [k_wave] -> X4/10(k_wave)
  [time] -> X4/1(time)
  Constant10/1 -> XB/4(vert2)
  [A_wave] -> Subsystem/9(A_wave)
  Add/1 -> Out1/1
  Constant103/1 -> Subsystem/4(vert2)
  Constant3/1 -> Subsystem/28(vert12)
  [g] -> XB/13(g)
  Constant42/1 -> X3/5(vert3)
  Constant58/1 -> X4/3(vert1)
  Constant5/1 -> Subsystem/31(normal3)
  [A_wave] -> X3/8(A_wave)
  Zb/1 -> [Zb]
  Constant6/1 -> Gain1/1
  Gain1/1 -> X1/19(EAX)
  dX_CTRL/1 -> Selector2/1, Selector3/1, Selector5/1, Selector4/1, Selector1/1
  Selector1/1 -> [dX1]
  Selector2/1 -> [dX2]
  Selector3/1 -> [dX3]
  Selector4/1 -> [dX4]
  Selector5/1 -> [dXB]
  [dX1] -> Gain2/1
  Gain2/1 -> X1/20(dX)
  Constant15/1 -> X1/21(Root_o)
  Constant70/1 -> Gain3/1
  Gain3/1 -> X2/20(EAX)
  [dX2] -> Gain4/1
  Gain4/1 -> X2/21(dX)
  Constant71/1 -> X2/22(Root_o)
  Gain5/1 -> X3/19(EAX)
  [dX3] -> Gain6/1
  Constant72/1 -> Gain5/1
  Gain6/1 -> X3/20(dX)
  Constant73/1 -> X3/21(Root_o)
  Constant75/1 -> X4/22(Root_o)
  Gain7/1 -> X4/20(EAX)
  Constant74/1 -> Gain7/1
  [dX4] -> Gain8/1
  Gain8/1 -> X4/21(dX)
  Constant77/1 -> Gain9/1
  Gain9/1 -> XB/21(EAX)
  [dXB] -> Gain10/1
  Constant76/1 -> XB/23(Root_o)
  Gain10/1 -> XB/22(dX)
  X4/1(Out1) -> Add/6
  X3/1(Out1) -> Add/5
  X2/1(Out1) -> Add/4
  X1/1(Out1) -> Add/3
  XB/1(Out1) -> Add/2
  Subsystem/1(Out1) -> Add/1

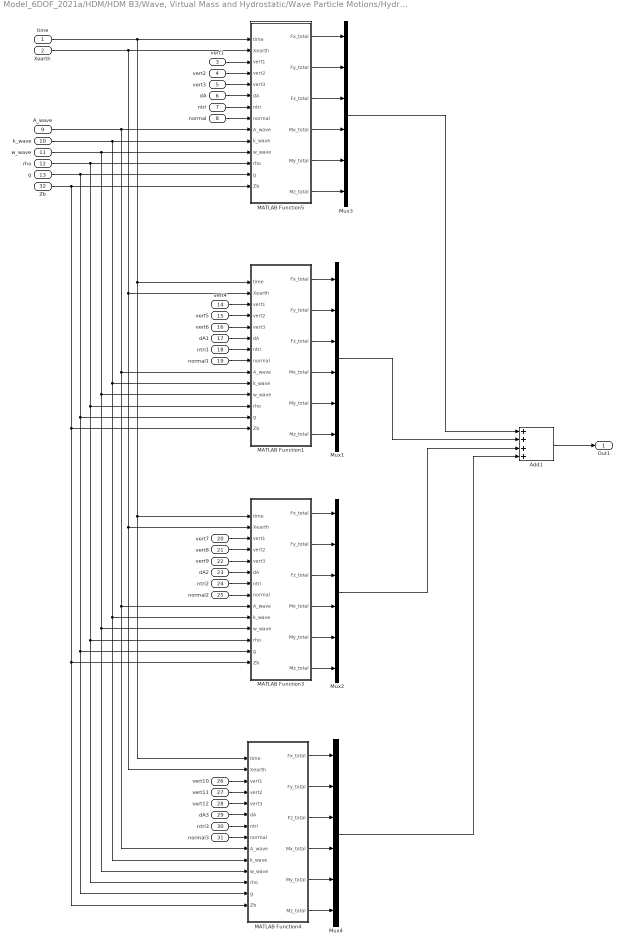
== system Model_6DOF_2021a/HDM/HDM B3/Wave, Virtual Mass and Hydrostatic/Wave Particle Motions/Hydrostatic Forces and Moments/Subsystem ==
  time : Inport
  Xearth : Inport  Port=2
  vert1 : Inport  Port=3
  vert2 : Inport  Port=4
  vert3 : Inport  Port=5
  dA : Inport  Port=6
  ntri : Inport  Port=7
  normal : Inport  Port=8
  A_wave : Inport  Port=9
  k_wave : Inport  Port=10
  w_wave : Inport  Port=11
  rho : Inport  Port=12
  g : Inport  Port=13
  vert4 : Inport  Port=14
  vert5 : Inport  Port=15
  vert6 : Inport  Port=16
  dA1 : Inport  Port=17
  ntri1 : Inport  Port=18
  normal1 : Inport  Port=19
  vert7 : Inport  Port=20
  vert8 : Inport  Port=21
  vert9 : Inport  Port=22
  dA2 : Inport  Port=23
  ntri2 : Inport  Port=24
  normal2 : Inport  Port=25
  vert10 : Inport  Port=26
  vert11 : Inport  Port=27
  vert12 : Inport  Port=28
  dA3 : Inport  Port=29
  ntri3 : Inport  Port=30
  normal3 : Inport  Port=31
  Zb : Inport  Port=32
  Add1 : Sum  Inputs=4
  MATLAB Function1 : MATLAB Function  TreatAsAtomicUnit=on
  MATLAB Function3 : MATLAB Function  TreatAsAtomicUnit=on
  MATLAB Function4 : MATLAB Function  TreatAsAtomicUnit=on
  MATLAB Function5 : MATLAB Function  TreatAsAtomicUnit=on
  Mux{1..4} (4 alike) : Mux  Inputs=6
  Out1 : Outport
  wires:
  ntri1/1 -> MATLAB Function1/7(ntri)
  rho/1 -> MATLAB Function5/12(rho), MATLAB Function1/12(rho), MATLAB Function4/12(rho), MATLAB Function3/12(rho)
  vert5/1 -> MATLAB Function1/4(vert2)
  MATLAB Function5/5(My_total) -> Mux3/5
  time/1 -> MATLAB Function5/1(time), MATLAB Function1/1(time), MATLAB Function4/1(time), MATLAB Function3/1(time)
  Xearth/1 -> MATLAB Function5/2(Xearth), MATLAB Function4/2(Xearth), MATLAB Function3/2(Xearth), MATLAB Function1/2(Xearth)
  vert7/1 -> MATLAB Function3/3(vert1)
  MATLAB Function5/4(Mx_total) -> Mux3/4
  Mux3/1 -> Add1/1
  normal1/1 -> MATLAB Function1/8(normal)
  A_wave/1 -> MATLAB Function5/9(A_wave), MATLAB Function1/9(A_wave), MATLAB Function4/9(A_wave), MATLAB Function3/9(A_wave)
  MATLAB Function5/3(Fz_total) -> Mux3/3
  k_wave/1 -> MATLAB Function5/10(k_wave), MATLAB Function1/10(k_wave), MATLAB Function4/10(k_wave), MATLAB Function3/10(k_wave)
  w_wave/1 -> MATLAB Function5/11(w_wave), MATLAB Function1/11(w_wave), MATLAB Function4/11(w_wave), MATLAB Function3/11(w_wave)
  MATLAB Function5/2(Fy_total) -> Mux3/2
  ntri/1 -> MATLAB Function5/7(ntri)
  g/1 -> MATLAB Function5/13(g), MATLAB Function1/13(g), MATLAB Function4/13(g), MATLAB Function3/13(g)
  dA2/1 -> MATLAB Function3/6(dA)
  MATLAB Function5/1(Fx_total) -> Mux3/1
  vert12/1 -> MATLAB Function4/5(vert3)
  normal3/1 -> MATLAB Function4/8(normal)
  vert4/1 -> MATLAB Function1/3(vert1)
  vert9/1 -> MATLAB Function3/5(vert3)
  normal/1 -> MATLAB Function5/8(normal)
  dA/1 -> MATLAB Function5/6(dA)
  MATLAB Function5/6(Mz_total) -> Mux3/6
  vert11/1 -> MATLAB Function4/4(vert2)
  ntri2/1 -> MATLAB Function3/7(ntri)
  ntri3/1 -> MATLAB Function4/7(ntri)
  dA3/1 -> MATLAB Function4/6(dA)
  vert2/1 -> MATLAB Function5/4(vert2)
  Add1/1 -> Out1/1
  vert6/1 -> MATLAB Function1/5(vert3)
  vert3/1 -> MATLAB Function5/5(vert3)
  normal2/1 -> MATLAB Function3/8(normal)
  dA1/1 -> MATLAB Function1/6(dA)
  vert10/1 -> MATLAB Function4/3(vert1)
  vert1/1 -> MATLAB Function5/3(vert1)
  vert8/1 -> MATLAB Function3/4(vert2)
  Zb/1 -> MATLAB Function5/14(Zb), MATLAB Function1/14(Zb), MATLAB Function3/14(Zb), MATLAB Function4/14(Zb)
  Mux2/1 -> Add1/3
  MATLAB Function1/6(Mz_total) -> Mux1/6
  Mux1/1 -> Add1/2
  MATLAB Function1/1(Fx_total) -> Mux1/1
  MATLAB Function1/2(Fy_total) -> Mux1/2
  MATLAB Function1/3(Fz_total) -> Mux1/3
  MATLAB Function1/4(Mx_total) -> Mux1/4
  MATLAB Function1/5(My_total) -> Mux1/5
  MATLAB Function3/5(My_total) -> Mux2/5
  MATLAB Function3/4(Mx_total) -> Mux2/4
  MATLAB Function3/3(Fz_total) -> Mux2/3
  MATLAB Function3/2(Fy_total) -> Mux2/2
  MATLAB Function3/1(Fx_total) -> Mux2/1
  MATLAB Function3/6(Mz_total) -> Mux2/6
  MATLAB Function4/6(Mz_total) -> Mux4/6
  MATLAB Function4/1(Fx_total) -> Mux4/1
  MATLAB Function4/2(Fy_total) -> Mux4/2
  MATLAB Function4/3(Fz_total) -> Mux4/3
  MATLAB Function4/4(Mx_total) -> Mux4/4
  MATLAB Function4/5(My_total) -> Mux4/5
  Mux4/1 -> Add1/4

== system Model_6DOF_2021a/HDM/HDM B3/Wave, Virtual Mass and Hydrostatic/Wave Particle Motions/Hydrostatic Forces and Moments/X1 ==
  time : Inport
  Xearth : Inport  Port=2
  vert1 : Inport  Port=3
  vert2 : Inport  Port=4
  vert3 : Inport  Port=5
  dA : Inport  Port=6
  ntri : Inport  Port=7
  A_wave : Inport  Port=8
  k_wave : Inport  Port=9
  w_wave : Inport  Port=10
  rho : Inport  Port=11
  g : Inport  Port=12
  vert4 : Inport  Port=13
  vert5 : Inport  Port=14
  vert6 : Inport  Port=15
  dA1 : Inport  Port=16
  ntri1 : Inport  Port=17
  Zb : Inport  Port=18
  EAX : Inport  Port=19
  dX : Inport  Port=20
  Root_o : Inport  Port=21
  Add1 : Sum
  CG : Constant  Value=[32.3114; 0; 0;]
  MATLAB Function1 : MATLAB Function  TreatAsAtomicUnit=on
  MATLAB Function4 : MATLAB Function  TreatAsAtomicUnit=on
  Mux1 : Mux  Inputs=6
  Mux2 : Mux  Inputs=6
  Out1 : Outport
  wires:
  ntri1/1 -> MATLAB Function1/7(ntri)
  dA1/1 -> MATLAB Function1/6(dA)
  vert6/1 -> MATLAB Function1/5(vert3)
  vert5/1 -> MATLAB Function1/4(vert2)
  vert4/1 -> MATLAB Function1/3(vert1)
  Zb/1 -> MATLAB Function1/13(Zb), MATLAB Function4/13(Zb)
  vert2/1 -> MATLAB Function4/4(vert2)
  ntri/1 -> MATLAB Function4/7(ntri)
  time/1 -> MATLAB Function4/1(time), MATLAB Function1/1(time)
  vert1/1 -> MATLAB Function4/3(vert1)
  Mux1/1 -> Add1/2
  vert3/1 -> MATLAB Function4/5(vert3)
  Mux2/1 -> Add1/1
  MATLAB Function4/2(Fy_total) -> Mux2/2
  MATLAB Function4/6(Mz_total) -> Mux2/6
  g/1 -> MATLAB Function1/12(g), MATLAB Function4/12(g)
  k_wave/1 -> MATLAB Function4/9(k_wave), MATLAB Function1/9(k_wave)
  dA/1 -> MATLAB Function4/6(dA)
  MATLAB Function4/5(My_total) -> Mux2/5
  MATLAB Function1/3(Fz_total) -> Mux1/3
  Add1/1 -> Out1/1
  MATLAB Function1/1(Fx_total) -> Mux1/1
  MATLAB Function4/1(Fx_total) -> Mux2/1
  MATLAB Function1/4(Mx_total) -> Mux1/4
  A_wave/1 -> MATLAB Function1/8(A_wave), MATLAB Function4/8(A_wave)
  rho/1 -> MATLAB Function1/11(rho), MATLAB Function4/11(rho)
  Xearth/1 -> MATLAB Function4/2(Xearth), MATLAB Function1/2(Xearth)
  MATLAB Function1/2(Fy_total) -> Mux1/2
  w_wave/1 -> MATLAB Function1/10(w_wave), MATLAB Function4/10(w_wave)
  MATLAB Function4/4(Mx_total) -> Mux2/4
  MATLAB Function4/3(Fz_total) -> Mux2/3
  EAX/1 -> MATLAB Function1/14(EAX), MATLAB Function4/14(EAX)
  dX/1 -> MATLAB Function4/15(dX), MATLAB Function1/15(dX)
  Root_o/1 -> MATLAB Function1/16(origin), MATLAB Function4/16(origin)
  CG/1 -> MATLAB Function1/17(xcg), MATLAB Function4/17(xcg)
  MATLAB Function1/5(My_total) -> Mux1/5
  MATLAB Function1/6(Mz_total) -> Mux1/6

== system Model_6DOF_2021a/HDM/HDM B3/Wave, Virtual Mass and Hydrostatic/Wave Particle Motions/Hydrostatic Forces and Moments/X2 ==
  time : Inport
  Xearth : Inport  Port=2
  vert1 : Inport  Port=3
  vert2 : Inport  Port=4
  vert3 : Inport  Port=5
  dA : Inport  Port=6
  ntri : Inport  Port=7
  normal : Inport  Port=8
  A_wave : Inport  Port=9
  k_wave : Inport  Port=10
  w_wave : Inport  Port=11
  rho : Inport  Port=12
  g : Inport  Port=13
  vert4 : Inport  Port=14
  vert5 : Inport  Port=15
  vert6 : Inport  Port=16
  dA1 : Inport  Port=17
  ntri1 : Inport  Port=18
  Zb : Inport  Port=19
  EAX : Inport  Port=20
  dX : Inport  Port=21
  Root_o : Inport  Port=22
  Add1 : Sum
  CG : Constant  Value=[32.3114; 0; 0;]
  MATLAB Function1 : MATLAB Function  TreatAsAtomicUnit=on
  MATLAB Function4 : MATLAB Function  TreatAsAtomicUnit=on
  Mux1 : Mux  Inputs=6
  Mux2 : Mux  Inputs=6
  Out1 : Outport
  wires:
  MATLAB Function1/6(Mz_total) -> Mux1/6
  MATLAB Function1/5(My_total) -> Mux1/5
  CG/1 -> MATLAB Function1/17(xcg), MATLAB Function4/17(xcg)
  Root_o/1 -> MATLAB Function1/16(origin), MATLAB Function4/16(origin)
  dX/1 -> MATLAB Function1/15(dX), MATLAB Function4/15(dX)
  EAX/1 -> MATLAB Function1/14(EAX), MATLAB Function4/14(EAX)
  MATLAB Function4/3(Fz_total) -> Mux2/3
  MATLAB Function4/4(Mx_total) -> Mux2/4
  w_wave/1 -> MATLAB Function1/10(w_wave), MATLAB Function4/10(w_wave)
  MATLAB Function1/2(Fy_total) -> Mux1/2
  Xearth/1 -> MATLAB Function1/2(Xearth), MATLAB Function4/2(Xearth)
  rho/1 -> MATLAB Function1/11(rho), MATLAB Function4/11(rho)
  A_wave/1 -> MATLAB Function1/8(A_wave), MATLAB Function4/8(A_wave)
  MATLAB Function1/4(Mx_total) -> Mux1/4
  MATLAB Function4/1(Fx_total) -> Mux2/1
  MATLAB Function1/1(Fx_total) -> Mux1/1
  Add1/1 -> Out1/1
  MATLAB Function1/3(Fz_total) -> Mux1/3
  MATLAB Function4/5(My_total) -> Mux2/5
  dA/1 -> MATLAB Function4/6(dA)
  k_wave/1 -> MATLAB Function1/9(k_wave), MATLAB Function4/9(k_wave)
  g/1 -> MATLAB Function1/12(g), MATLAB Function4/12(g)
  MATLAB Function4/6(Mz_total) -> Mux2/6
  MATLAB Function4/2(Fy_total) -> Mux2/2
  Mux2/1 -> Add1/1
  vert3/1 -> MATLAB Function4/5(vert3)
  Mux1/1 -> Add1/2
  vert1/1 -> MATLAB Function4/3(vert1)
  time/1 -> MATLAB Function1/1(time), MATLAB Function4/1(time)
  normal/1 -> ?
  ntri/1 -> MATLAB Function4/7(ntri)
  vert2/1 -> MATLAB Function4/4(vert2)
  Zb/1 -> MATLAB Function1/13(Zb), MATLAB Function4/13(Zb)
  vert4/1 -> MATLAB Function1/3(vert1)
  vert5/1 -> MATLAB Function1/4(vert2)
  vert6/1 -> MATLAB Function1/5(vert3)
  dA1/1 -> MATLAB Function1/6(dA)
  ntri1/1 -> MATLAB Function1/7(ntri)
